simulink model "QuadcopterSimModel_INDI_Traj"  (R2018b)
settings: Solver=ode23  StartTime=0.0  StopTime=1000  FixedStep=sample_time  RelTol=1e-4  EnableMultiTasking=on
undefined symbols (not defined in the file): alt_ground, atmosphere, cycle, DiscIntNeverNeededParam, envir, fm_loiter, g, jystck, pos_ref, sigbuilder_block, traj_empty, waypoints, wind
libraries: simulink x6, ndi_lib x5, filters_lib x5, axes_transformation_lib x4, angles_lib x3, unit_conversions_lib x3, cntrl_atti_red_indi_lib x2, traj_lib x2, aerolibfltsims x2, control_allocation_lib x1, sensors_lib x1, atmosphere_lib x1
(part 2 of 3)

== system QuadcopterSimModel_INDI_Traj/stick inputs/Signal builder/Signal Builder2 ==
  Demux : Demux  Tag=STV Demux  Outputs=1
  FromWs : FromWorkspace  Tag=STV FromWs  VariableName=tuvar  SampleTime=0
      SigBuilderData=|
      | common.afterFinalStr = 'Extrapolate'
      | common.sampleTime = 0
      | dataSet.timeRange = [0 10]
      | dataSet.name = 'Group 1'
      | sbobj.Groups.Name = 'Group 1'
      | sbobj.Groups.Signals.Name = 'Signal 1'
      | sbobj.Groups.Signals.XData = [0 2 2 6 8 10]
      | sbobj.Groups.Signals.YData = [0 0 -1 -1 0 0]
  Signal 1 : Outport  Tag=STV Outport
  wires:
  FromWs/1 -> Demux/1
  Demux/1 -> Signal 1/1

== system QuadcopterSimModel_INDI_Traj/stick inputs/Signal builder/Signal Builder3 ==
  Demux : Demux  Tag=STV Demux  Outputs=1
  FromWs : FromWorkspace  Tag=STV FromWs  VariableName=tuvar  SampleTime=0
      SigBuilderData=|
      | common.afterFinalStr = 'Extrapolate'
      | common.sampleTime = 0
      | dataSet.timeRange = [0 10]
      | dataSet.name = 'Group 1'
      | sbobj.Groups.Name = 'Group 1'
      | sbobj.Groups.Signals.Name = 'Signal 1'
      | sbobj.Groups.Signals.XData = [0 6 6 8 8 10]
      | sbobj.Groups.Signals.YData = [0 0 1 1 0 0]
  Signal 1 : Outport  Tag=STV Outport
  wires:
  Demux/1 -> Signal 1/1
  FromWs/1 -> Demux/1

== system QuadcopterSimModel_INDI_Traj/Controller INDI/Multicopter INDI Loiter Flight Mode/Delta attitude to stick commands/conversion to total attitude command ==
  Delta_q : Inport
  Delta_n_g : Inport  Port=2
  M_bg : Inport  Port=3
  Add : Sum
  DCM to quaternions : axes_transformation_lib/DCM to quaternions  SystemSampleTime=-1
      settings: SourceProductName=LADAC
  MATLAB Function : MATLAB Function  TreatAsAtomicUnit=on
  MATLAB Function1 : MATLAB Function  TreatAsAtomicUnit=on
  MATLAB Function4 : MATLAB Function  TreatAsAtomicUnit=on
  Scope : Scope  NumInputPorts=4
  quaternion to lean angles : Subsystem
  total reduced attitude command (quaternion) : MATLAB Function  TreatAsAtomicUnit=on
  lean_angle : Outport
  lean_direction_angle : Outport  Port=2
  wires:
  DCM to quaternions/1 -> total reduced attitude command (quaternion)/2(q_m)
  M_bg/1 -> MATLAB Function1/1(M_bg), DCM to quaternions/1
  quaternion to lean angles/1(phi) -> Scope/1
  total reduced attitude command (quaternion)/1(q_cmd) -> quaternion to lean angles/1(q_bg)
  Add/1 -> MATLAB Function/1(u)
  Delta_q/1 -> total reduced attitude command (quaternion)/1(q_e)
  MATLAB Function4/1(phi) -> lean_angle/1, Scope/3
  quaternion to lean angles/2(delta) -> Scope/2
  MATLAB Function4/2(delta) -> Scope/4, lean_direction_angle/1
  Delta_n_g/1 -> Add/1
  MATLAB Function1/1(n_g) -> Add/2
  MATLAB Function/1(y) -> MATLAB Function4/1(n_g)

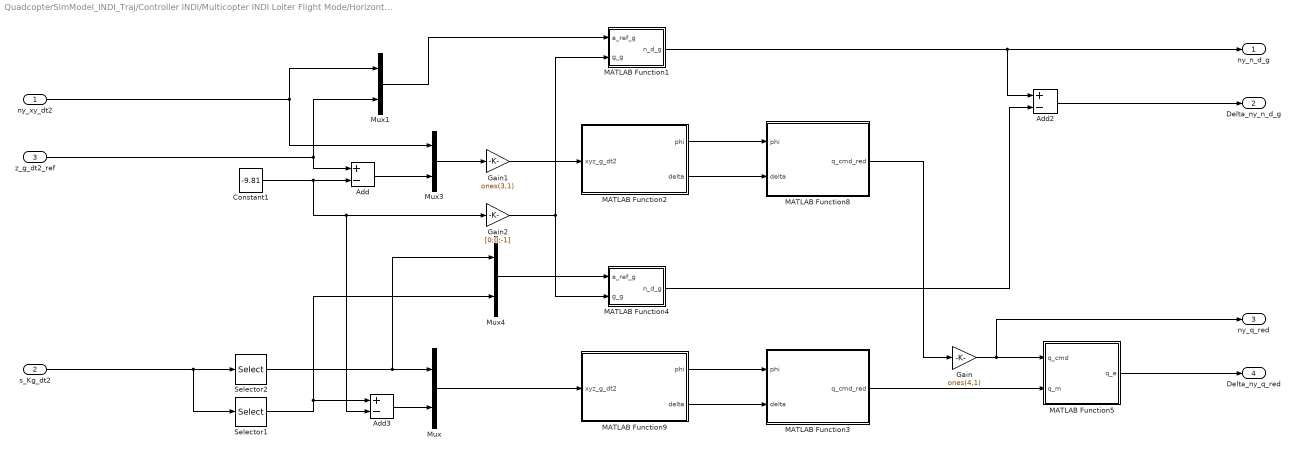
== system QuadcopterSimModel_INDI_Traj/Controller INDI/Multicopter INDI Loiter Flight Mode/Horizontal NDI position (NE) controller cascade with reduced attitude (angle) command/Convert to reduced attitude pseudo control ==
  ny_xy_dt2 : Inport
  s_Kg_dt2 : Inport  Port=2
  z_g_dt2_ref : Inport  Port=3
  Add : Sum  Inputs=+-
  Add2 : Sum  Inputs=+-
  Add3 : Sum  Inputs=+-
  Constant1 : Constant  Value=-9.81  OutDataTypeStr=single
  Gain : Gain  Gain=ones(4,1)
  Gain1 : Gain  Gain=ones(3,1)
  Gain2 : Gain  Gain=[0;0;-1]
  MATLAB Function1 : MATLAB Function  TreatAsAtomicUnit=on
  MATLAB Function2 : MATLAB Function  TreatAsAtomicUnit=on
  MATLAB Function3 : MATLAB Function  TreatAsAtomicUnit=on
  MATLAB Function4 : MATLAB Function  TreatAsAtomicUnit=on
  MATLAB Function5 : MATLAB Function  TreatAsAtomicUnit=on
  MATLAB Function8 : MATLAB Function  TreatAsAtomicUnit=on
  MATLAB Function9 : MATLAB Function  TreatAsAtomicUnit=on
  Mux{,1,3..4} (4 alike) : Mux  Inputs=2
  Selector1 : Selector  InputPortWidth=3  IndexOptions=Index vector (dialog)  Indices=3  OutputSizes=1
  Selector2 : Selector  InputPortWidth=3  IndexOptions=Index vector (dialog)  Indices=[1,2]  OutputSizes=1
  ny_n_d_g : Outport
  Delta_ny_n_d_g : Outport  Port=2
  ny_q_red : Outport  Port=3
  Delta_ny_q_red : Outport  Port=4
  wires:
  MATLAB Function2/1(phi) -> MATLAB Function8/1(phi)
  MATLAB Function8/1(q_cmd_red) -> Gain/1
  Gain/1 -> MATLAB Function5/1(q_cmd), ny_q_red/1
  MATLAB Function1/1(n_d_g) -> Add2/1, ny_n_d_g/1
  Constant1/1 -> Add3/2, Gain2/1, Add/2
  Mux3/1 -> Gain1/1
  ny_xy_dt2/1 -> Mux1/1, Mux3/1
  Mux1/1 -> MATLAB Function1/1(a_ref_g)
  MATLAB Function5/1(q_e) -> Delta_ny_q_red/1
  MATLAB Function9/1(phi) -> MATLAB Function3/1(phi)
  Gain2/1 -> MATLAB Function4/2(g_g), MATLAB Function1/2(g_g)
  Mux4/1 -> MATLAB Function4/1(a_ref_g)
  Add2/1 -> Delta_ny_n_d_g/1
  z_g_dt2_ref/1 -> Mux1/2, Add/1
  Gain1/1 -> MATLAB Function2/1(xyz_g_dt2)
  Add/1 -> Mux3/2
  MATLAB Function9/2(delta) -> MATLAB Function3/2(delta)
  s_Kg_dt2/1 -> Selector2/1, Selector1/1
  Add3/1 -> Mux/2
  Selector2/1 -> Mux4/1, Mux/1
  MATLAB Function4/1(n_d_g) -> Add2/2
  Selector1/1 -> Add3/1, Mux4/2
  MATLAB Function3/1(q_cmd_red) -> MATLAB Function5/2(q_m)
  MATLAB Function2/2(delta) -> MATLAB Function8/2(delta)
  Mux/1 -> MATLAB Function9/1(xyz_g_dt2)

== system QuadcopterSimModel_INDI_Traj/Controller INDI/Multicopter INDI Loiter Flight Mode/Horizontal NDI position (NE) controller cascade with reduced attitude (angle) command/filtered command ==
  cmd_forward_velocity_-1_1 : Inport
  cmd_lateral_velocity_-1_1 : Inport  Port=2
  initial_horizontal_position : Inport  Port=3
  manual_mode : Inport  Port=4
  Bus Creator : BusCreator  Inputs=3
  Bus Selector2 : BusSelector  OutputSignals=x_ref,x_dt_ref
  Discrete-Time Integrator : DiscreteIntegrator  ExternalReset=rising  InitialConditionSource=external  SampleTime=-1  ICPrevOutput=DiscIntNeverNeededParam  ICPrevScaledInput=DiscIntNeverNeededParam
  Gain : Gain
  Gain1 : Gain
  Gain3 : Gain  Gain=horiz_pos_cntrl.rm.uv_max
  MATLAB Function1 : MATLAB Function  TreatAsAtomicUnit=on
  Mux : Mux  Inputs=2
  PT1 discrete reference model : ndi_lib/PT1 discrete reference model  T=horiz_pos_cntrl.rm.uv_T  x_max=inf  x_min=-inf  x_dt_max=horiz_pos_cntrl.rm.uv_dt_max  x_dt_min=-horiz_pos_cntrl.rm.uv_dt_max  x_init=0
      settings: SourceProductName=LADAC
  Product : Product
  Terminator : Terminator
  ny : Outport
  reference : Outport  Port=2
  wires:
  Gain3/1 -> Product/2
  Product/1 -> PT1 discrete reference model/1
  MATLAB Function1/1(cmd_velocity_abs_0_1) -> Gain3/1
  MATLAB Function1/2(lean_direction_angle) -> Terminator/1
  Mux/1 -> Product/1
  Gain1/1 -> Bus Creator/3, ny/1  "xy_g_dt2"
  Gain/1 -> Bus Creator/2  "xy_g_dt"
  cmd_lateral_velocity_-1_1/1 -> MATLAB Function1/1(stick_roll_cmd), Mux/2
  initial_horizontal_position/1 -> Discrete-Time Integrator/3
  Bus Selector2/2 -> Gain1/1  "<x_dt_ref>"
  Bus Selector2/1 -> Discrete-Time Integrator/1, Gain/1  "<x_ref>"
  Discrete-Time Integrator/1 -> Bus Creator/1  "xy_g"
  PT1 discrete reference model/1 -> Bus Selector2/1
  Bus Creator/1 -> reference/1
  cmd_forward_velocity_-1_1/1 -> MATLAB Function1/2(stick_pitch_cmd), Mux/1
  manual_mode/1 -> Discrete-Time Integrator/2

== system QuadcopterSimModel_INDI_Traj/Controller INDI/Multicopter INDI Loiter Flight Mode/Horizontal NDI position (NE) controller cascade with reduced attitude (angle) command/measures ==
  xy_g : Inport
  xy_g_dt : Inport  Port=2
  s_Kg_dt2 : Inport  Port=3
  Bus Creator1 : BusCreator  Inputs=4
  Selector3 : Selector  InputPortWidth=3  IndexOptions=Index vector (dialog)  Indices=[1,2]  OutputSizes=1
  Selector4 : Selector  InputPortWidth=3  IndexOptions=Index vector (dialog)  Indices=[1,2]  OutputSizes=1
  Selector5 : Selector  InputPortWidth=3  IndexOptions=Index vector (dialog)  Indices=[1,2]  OutputSizes=1
  Selector6 : Selector  InputPortWidth=3  IndexOptions=Index vector (dialog)  Indices=3  OutputSizes=1
  measure : Outport
  wires:
  s_Kg_dt2/1 -> Selector6/1, Selector5/1
  xy_g_dt/1 -> Selector4/1
  xy_g/1 -> Selector3/1
  Selector4/1 -> Bus Creator1/2  "xy_g_dt"
  Selector3/1 -> Bus Creator1/1  "xy_g"
  Selector5/1 -> Bus Creator1/3  "xy_g_dt2"
  Selector6/1 -> Bus Creator1/4  "z_g_dt2"
  Bus Creator1/1 -> measure/1

== system QuadcopterSimModel_INDI_Traj/Controller INDI/Multicopter INDI Loiter Flight Mode/Horizontal NDI position (NE) controller cascade with reduced attitude (angle) command/position controller ==
  reference : Inport
  measure : Inport  Port=2
  Add : Sum  Inputs=+-
  Bus Selector : BusSelector  OutputSignals=xy_g,xy_g_dt,xy_g_dt2
  Bus to Vector : BusToVector
  Gain : Gain  Gain=horiz_pos_cntrl.K  Multiplication=Matrix(K*u)
  Mux : Mux  Inputs=3
  PT2 discrete with saturation : filters_lib/PT2 discrete with saturation  omega=2./T  d=1  x_dt2_max=inf  x_dt2_min=-inf  x_dt_max=inf  x_dt_min=-inf  x_max=inf  x_min=-inf  x_init=0  x_dt_init=0
      settings: SourceProductName=LADAC
  Saturation : Saturate  UpperLimit=horiz_pos_cntrl.limits.uv_dt_max  LowerLimit=-horiz_pos_cntrl.limits.uv_dt_max
  Saturation1 : Saturate  UpperLimit=[horiz_pos_cntrl.limits.e_xy_max;1000;1000;1000;1000]  LowerLimit=-[horiz_pos_cntrl.limits.e_xy_max;1000;1000;1000;1000]
  Terminator : Terminator
  Terminator1 : Terminator
  ny_cntrl : Outport
  e : Outport  Port=2
  wires:
  PT2 discrete with saturation/1 -> Add/1
  PT2 discrete with saturation/3 -> Terminator1/1
  PT2 discrete with saturation/2 -> Terminator/1
  Bus to Vector/1 -> PT2 discrete with saturation/1
  Bus Selector/1 -> Mux/1  "<xy_g>"
  Bus Selector/2 -> Mux/2  "<xy_g_dt>"
  Bus Selector/3 -> Mux/3  "<xy_g_dt2>"
  Mux/1 -> Add/2
  measure/1 -> Bus Selector/1
  Gain/1 -> Saturation/1
  Saturation1/1 -> Gain/1
  Saturation/1 -> ny_cntrl/1
  Add/1 -> e/1, Saturation1/1
  reference/1 -> Bus to Vector/1

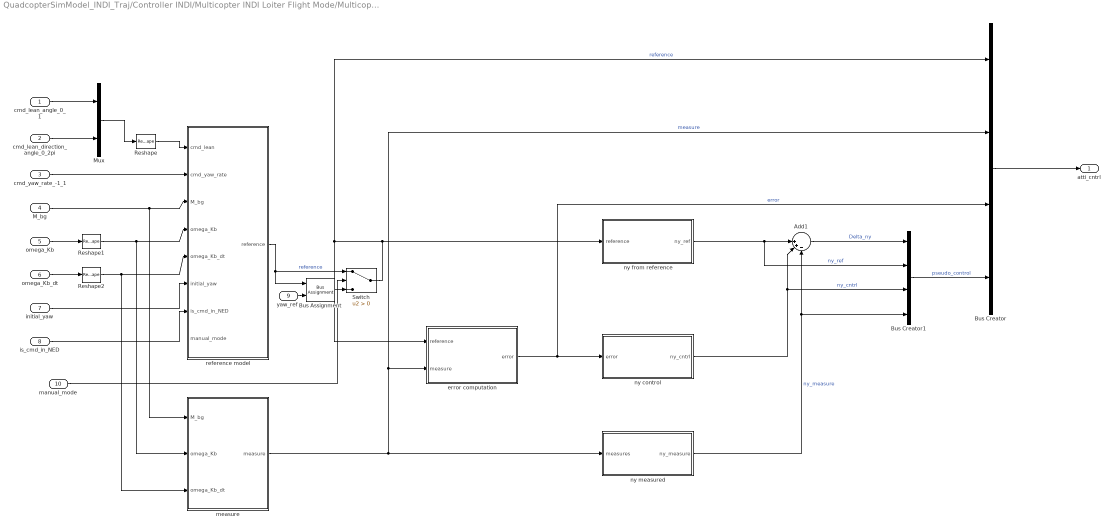
== system QuadcopterSimModel_INDI_Traj/Controller INDI/Multicopter INDI Loiter Flight Mode/Multicopter Altitude Hold Flight Mode with INDI and reduced attitude control/Multicopter (Reduced) Attitude INDI Controller ==
  cmd_lean_angle_0_1 : Inport
  cmd_lean_direction_angle_0_2pi : Inport  Port=2
  cmd_yaw_rate_-1_1 : Inport  Port=3
  M_bg : Inport  Port=4
  omega_Kb : Inport  Port=5
  omega_Kb_dt : Inport  Port=6
  initial_yaw : Inport  Port=7
  is_cmd_in_NED : Inport  Port=8
  "yaw_ref " : Inport  Port=9
  manual_mode : Inport  Port=10
  Add1 : Sum  Inputs=||++-
  Bus Assignment : BusAssignment  AssignedSignals=yaw
  Bus Creator : BusCreator  Inputs=4
  Bus Creator1 : BusCreator  Inputs=4
  Mux : Mux  Inputs=2
  Reshape : Reshape  OutputDimensionality=Column vector (2-D)
  Reshape1 : Reshape  OutputDimensionality=Column vector (2-D)
  Reshape2 : Reshape  OutputDimensionality=Column vector (2-D)
  Switch : Switch  Criteria=u2 > Threshold
  error computation : Subsystem
  measure : Subsystem
  ny control : Subsystem
  ny from reference : Subsystem
  ny measured : Subsystem
  reference model : Subsystem
  atti_cntrl : Outport
  wires:
  is_cmd_in_NED/1 -> reference model/7(is_cmd_in_NED)
  cmd_yaw_rate_-1_1/1 -> reference model/2(cmd_yaw_rate)
  cmd_lean_direction_angle_0_2pi/1 -> Mux/2
  cmd_lean_angle_0_1/1 -> Mux/1
  Reshape2/1 -> reference model/5(omega_Kb_dt), measure/3(omega_Kb_dt)
  Reshape1/1 -> reference model/4(omega_Kb), measure/2(omega_Kb)
  Reshape/1 -> reference model/1(cmd_lean)
  measure/1(measure) -> ny measured/1(measures), error computation/2(measure), Bus Creator/2  "measure"
  omega_Kb/1 -> Reshape1/1
  M_bg/1 -> reference model/3(M_bg), measure/1(M_bg)
  Add1/1 -> Bus Creator1/1  "Delta_ny"
  Bus Creator1/1 -> Bus Creator/4  "pseudo_control"
  Bus Creator/1 -> atti_cntrl/1
  initial_yaw/1 -> reference model/6(initial_yaw)
  Switch/1 -> error computation/1(reference), Bus Creator/1, ny from reference/1(reference)  "reference"
  ny measured/1(ny_measure) -> Add1/3, Bus Creator1/4  "ny_measure"
  ny control/1(ny_cntrl) -> Add1/2, Bus Creator1/3  "ny_cntrl"
  omega_Kb_dt/1 -> Reshape2/1
  error computation/1(error) -> Bus Creator/3, ny control/1(error)  "error"
  Mux/1 -> Reshape/1
  ny from reference/1(ny_ref) -> Add1/1, Bus Creator1/2  "ny_ref"
  manual_mode/1 -> Switch/2
  "yaw_ref "/1 -> Bus Assignment/2
  reference model/1(reference) -> Switch/1, Bus Assignment/1  "reference"
  Bus Assignment/1 -> Switch/3

== system QuadcopterSimModel_INDI_Traj/Controller INDI/Multicopter INDI Loiter Flight Mode/Multicopter Altitude Hold Flight Mode with INDI and reduced attitude control/Multicopter Altitude INDI Controller1 ==
  cmd_throttle_-1_1 : Inport
  z_Kg : Inport  Port=2
  z_Kg_dt : Inport  Port=3
  z_Kg_dt2 : Inport  Port=4
  initial_z_Kg : Inport  Port=5
  z_Ref : Inport  Port=6
  manual_mode : Inport  Port=7
  Add1 : Sum  Inputs=||++-
  Bus Creator : BusCreator  Inputs=4
  Bus Creator1 : BusCreator  Inputs=4
  Switch : Switch  Criteria=u2 > Threshold
  error computation : Subsystem
  measure : Subsystem
  ny control : Subsystem
  ny from reference : Subsystem
  ny measured : Subsystem
  reference model : Subsystem
  alt_cntrl : Outport
  wires:
  cmd_throttle_-1_1/1 -> reference model/1(cmd_throttle)
  z_Kg/1 -> measure/1(z_Kg)
  z_Kg_dt/1 -> measure/2(z_Kg_dt)
  z_Kg_dt2/1 -> measure/3(z_Kg_dt2)
  measure/1(measure) -> error computation/2(measure), Bus Creator/2, ny measured/1(measures)  "measure"
  Add1/1 -> Bus Creator1/1  "Delta_ny"
  Bus Creator1/1 -> Bus Creator/4  "pseudo_control"
  Bus Creator/1 -> alt_cntrl/1
  initial_z_Kg/1 -> reference model/2(initial_altitude)
  Switch/1 -> Bus Creator/1, ny from reference/1(reference_alt), error computation/1(reference)  "reference"
  ny measured/1(ny_measure) -> Add1/3, Bus Creator1/4  "ny_measure"
  ny control/1(ny_cntrl) -> Add1/2, Bus Creator1/3  "ny_cntrl"
  error computation/1(error) -> Bus Creator/3, ny control/1(error_alt)  "error"
  ny from reference/1(ny_ref) -> Add1/1, Bus Creator1/2  "ny_ref"
  z_Ref/1 -> Switch/3  "reference"
  reference model/1(reference) -> Switch/1  "reference"
  manual_mode/1 -> Switch/2, reference model/3(manual_mode)

== system QuadcopterSimModel_INDI_Traj/Controller INDI/Multicopter INDI Loiter Flight Mode/Multicopter Altitude Hold Flight Mode with INDI and reduced attitude control/acceleration g to b frame ==
  z_Kg_dt2_cmd : Inport
  M_bg : Inport  Port=2
  MATLAB Function : MATLAB Function  TreatAsAtomicUnit=on
  dcm2Lean : MATLAB Function  TreatAsAtomicUnit=on
  z_Kb_dt2_cmd : Outport
  wires:
  dcm2Lean/1(phi) -> MATLAB Function/2(lean_angle)
  M_bg/1 -> dcm2Lean/1(M_bg)
  MATLAB Function/1(z_Kb_dt2_cmd) -> z_Kb_dt2_cmd/1
  z_Kg_dt2_cmd/1 -> MATLAB Function/1(z_Kg_dt2_cmd)

== system QuadcopterSimModel_INDI_Traj/Controller INDI/Multicopter INDI Loiter Flight Mode/Multicopter Altitude Hold Flight Mode with INDI and reduced attitude control/control effectiveness ==
  u : Inport
  Constant : Constant  Value=fm.cntrl_effect.u_trim  OutDataTypeStr=single
  Constant1 : Constant  Value=fm.ca.u_min  OutDataTypeStr=single
  Constant4 : Constant  Value=fm.sample_time  OutDataTypeStr=single
  MATLAB Function : MATLAB Function  TreatAsAtomicUnit=on
  Max : MinMax  Function=max  Inputs=2  OutDataTypeStr=Inherit: Inherit via back propagation
  ny_du_dt : Constant  Value=fm.cntrl_effect.ny_du_dt  OutDataTypeStr=single
  ny_du_red_trim : Constant  Value=fm.cntrl_effect.ny_du_red  OutDataTypeStr=single
  G1 : Outport
  G2 : Outport  Port=2
  wires:
  ny_du_red_trim/1 -> MATLAB Function/1(ny_du_red_trim)
  Constant4/1 -> MATLAB Function/5(T_s)
  Constant/1 -> MATLAB Function/3(u_trim)
  ny_du_dt/1 -> MATLAB Function/2(ny_du_dt_trim)
  u/1 -> Max/1
  Constant1/1 -> Max/2
  Max/1 -> MATLAB Function/4(u)
  MATLAB Function/1(G1) -> G1/1
  MATLAB Function/2(G2) -> G2/1

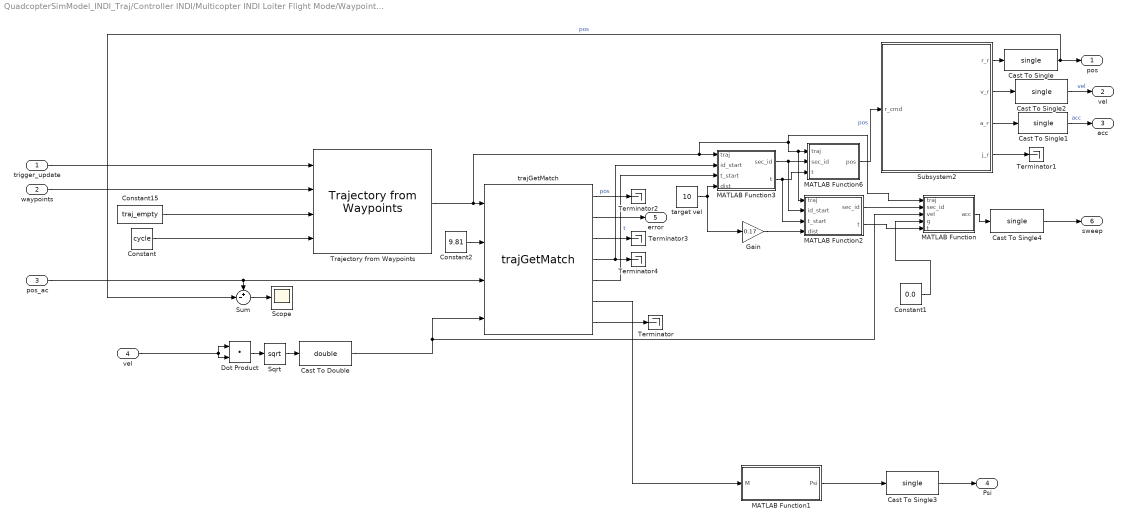
== system QuadcopterSimModel_INDI_Traj/Controller INDI/Multicopter INDI Loiter Flight Mode/Waypoint Reference/waypoint Reference System ==
  trigger_update : Inport
  waypoints : Inport  Port=2
  pos_ac : Inport  Port=3
  "vel " : Inport  Port=4
  Cast To Double : DataTypeConversion  OutDataTypeStr=double
  Cast To Single{,1..4} (5 alike) : DataTypeConversion  OutDataTypeStr=single
  Constant : Constant  Value=cycle
  Constant1 : Constant  Value=0.0
  Constant15 : Constant  Value=traj_empty  OutDataTypeStr=Bus: trajectoryBus
  Constant2 : Constant  Value=9.81
  Dot Product : DotProduct  InputSameDT=on  OutDataTypeStr=Inherit: Inherit via internal rule
  Gain : Gain  Gain=0.17
  MATLAB Function : MATLAB Function  TreatAsAtomicUnit=on
  MATLAB Function1 : MATLAB Function  TreatAsAtomicUnit=on
  MATLAB Function2 : MATLAB Function  TreatAsAtomicUnit=on
  MATLAB Function3 : MATLAB Function  TreatAsAtomicUnit=on
  MATLAB Function6 : MATLAB Function  TreatAsAtomicUnit=on
  Scope : Scope
  Sqrt : Sqrt  SaturateOnIntegerOverflow=on
  Subsystem2 : Subsystem
  Sum : Sum  Inputs=+-|
  Terminator{,1..4} (5 alike) : Terminator
  Trajectory from Waypoints : traj_lib/Trajectory from Waypoints
      settings: SourceProductName=LADAC
  target vel : Constant  Value=10
  trajGetMatch : traj_lib/trajGetMatch  SystemSampleTime=-1
      settings: SourceProductName=LADAC
  pos : Outport
  vel : Outport  Port=2
  acc : Outport  Port=3
  Psi : Outport  Port=4
  error : Outport  Port=5
  "sweep " : Outport  Port=6
  wires:
  Constant15/1 -> Trajectory from Waypoints/3
  waypoints/1 -> Trajectory from Waypoints/2
  trajGetMatch/4 -> MATLAB Function3/2(id_start), Terminator4/1
  "vel "/1 -> Dot Product/2, Dot Product/1
  Cast To Single1/1 -> acc/1  "acc"
  pos_ac/1 -> trajGetMatch/3, Sum/1
  Cast To Single2/1 -> vel/1  "vel"
  Cast To Single/1 -> Sum/2, pos/1  "pos"
  trajGetMatch/3 -> Terminator3/1
  Constant/1 -> Trajectory from Waypoints/4
  Constant2/1 -> trajGetMatch/2
  trajGetMatch/6 -> MATLAB Function1/1(M)
  trajGetMatch/5 -> MATLAB Function3/3(t_start)  "t"
  trigger_update/1 -> Trajectory from Waypoints/1
  trajGetMatch/2 -> error/1
  Cast To Single3/1 -> Psi/1
  MATLAB Function1/1(Psi) -> Cast To Single3/1
  Sum/1 -> Scope/1
  Dot Product/1 -> Sqrt/1
  Cast To Double/1 -> MATLAB Function/3(vel), trajGetMatch/4
  MATLAB Function3/1(sec_id) -> MATLAB Function2/2(id_start), MATLAB Function6/2(sec_id)
  Subsystem2/1(r_r) -> Cast To Single/1
  Subsystem2/2(v_r) -> Cast To Single2/1
  Subsystem2/3(a_r) -> Cast To Single1/1
  trajGetMatch/1 -> Terminator2/1  "pos"
  MATLAB Function6/1(pos) -> Subsystem2/1(r_cmd)  "pos"
  target vel/1 -> MATLAB Function3/4(dist), Gain/1
  Sqrt/1 -> Cast To Double/1
  trajGetMatch/7 -> Terminator/1
  Subsystem2/4(j_r) -> Terminator1/1
  MATLAB Function3/2(t) -> MATLAB Function2/3(t_start), MATLAB Function6/3(t)
  Gain/1 -> MATLAB Function2/4(dist)
  MATLAB Function2/2(t) -> MATLAB Function/5(t)
  MATLAB Function2/1(sec_id) -> MATLAB Function/2(sec_id)
  Constant1/1 -> MATLAB Function/4(g)
  MATLAB Function/1(acc) -> Cast To Single4/1
  Cast To Single4/1 -> "sweep "/1
  Trajectory from Waypoints/1 -> MATLAB Function/1(traj), MATLAB Function2/1(traj), MATLAB Function6/1(traj), MATLAB Function3/1(traj), trajGetMatch/1

== system QuadcopterSimModel_INDI_Traj/Controller INDI/Multicopter INDI Loiter Flight Mode/Delta attitude to stick commands/conversion to total attitude command/quaternion to lean angles ==
  q_bg : Inport
  MATLAB Function4 : MATLAB Function  TreatAsAtomicUnit=on
  quaternion to reduced attitude unit vector : MATLAB Function  TreatAsAtomicUnit=on
  phi : Outport
  delta : Outport  Port=2
  wires:
  MATLAB Function4/2(delta) -> delta/1
  q_bg/1 -> quaternion to reduced attitude unit vector/1(q_bg)
  MATLAB Function4/1(phi) -> phi/1
  quaternion to reduced attitude unit vector/1(n_g) -> MATLAB Function4/1(n_g)

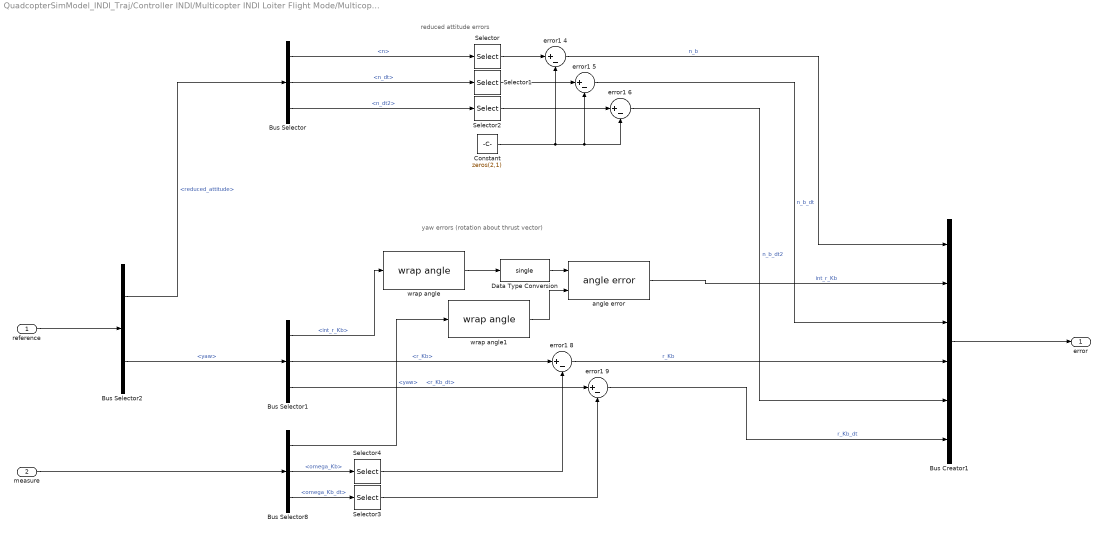
== system QuadcopterSimModel_INDI_Traj/Controller INDI/Multicopter INDI Loiter Flight Mode/Multicopter Altitude Hold Flight Mode with INDI and reduced attitude control/Multicopter (Reduced) Attitude INDI Controller/error computation ==
  note: yaw errors (rotation about thrust vector)
  note: reduced attitude errors
  reference : Inport
  measure : Inport  Port=2
  Bus Creator1 : BusCreator  Inputs=6
  Bus Selector : BusSelector  OutputSignals=n,n_dt,n_dt2
  Bus Selector1 : BusSelector  OutputSignals=int_r_Kb,r_Kb,r_Kb_dt
  Bus Selector2 : BusSelector  OutputSignals=reduced_attitude,yaw
  Bus Selector8 : BusSelector  OutputSignals=yaw,omega_Kb,omega_Kb_dt
  Constant : Constant  Value=zeros(2,1)  OutDataTypeStr=Inherit: Inherit via back propagation
  Data Type Conversion : DataTypeConversion  OutDataTypeStr=single
  Selector : Selector  InputPortWidth=3  IndexOptions=Index vector (dialog)  Indices=[1,2]  OutputSizes=1
  Selector1 : Selector  InputPortWidth=3  IndexOptions=Index vector (dialog)  Indices=[1,2]  OutputSizes=1
  Selector2 : Selector  InputPortWidth=3  IndexOptions=Index vector (dialog)  Indices=[1,2]  OutputSizes=1
  Selector3 : Selector  InputPortWidth=3  IndexOptions=Index vector (dialog)  Indices=3  OutputSizes=1
  Selector4 : Selector  InputPortWidth=3  IndexOptions=Index vector (dialog)  Indices=3  OutputSizes=1
  angle error : angles_lib/angle error  SystemSampleTime=-1
      settings: SourceProductName=LADAC
  error1 {4..6,8..9} (5 alike) : Sum  Inputs=|+-
  wrap angle : angles_lib/wrap angle  SystemSampleTime=-1
      settings: SourceProductName=LADAC
  wrap angle1 : angles_lib/wrap angle  SystemSampleTime=-1
      settings: SourceProductName=LADAC
  error : Outport
  wires:
  Data Type Conversion/1 -> angle error/1
  wrap angle/1 -> Data Type Conversion/1
  wrap angle1/1 -> angle error/2
  error1 9/1 -> Bus Creator1/6  "r_Kb_dt"
  error1 6/1 -> Bus Creator1/5  "n_b_dt2"
  error1 5/1 -> Bus Creator1/3  "n_b_dt"
  error1 8/1 -> Bus Creator1/4  "r_Kb"
  angle error/1 -> Bus Creator1/2  "int_r_Kb"
  Selector3/1 -> error1 9/2
  Selector4/1 -> error1 8/2
  Bus Selector8/1 -> wrap angle1/1  "<yaw>"
  Bus Selector8/2 -> Selector4/1  "<omega_Kb>"
  Bus Selector8/3 -> Selector3/1  "<omega_Kb_dt>"
  measure/1 -> Bus Selector8/1
  Bus Selector1/3 -> error1 9/1  "<r_Kb_dt>"
  Bus Selector1/2 -> error1 8/1  "<r_Kb>"
  Bus Selector1/1 -> wrap angle/1  "<int_r_Kb>"
  Bus Selector2/2 -> Bus Selector1/1  "<yaw>"
  Constant/1 -> error1 4/2, error1 5/2, error1 6/2
  Selector2/1 -> error1 6/1
  Selector1/1 -> error1 5/1
  Selector/1 -> error1 4/1
  Bus Creator1/1 -> error/1
  Bus Selector2/1 -> Bus Selector/1  "<reduced_attitude>"
  Bus Selector/3 -> Selector2/1  "<n_dt2>"
  Bus Selector/2 -> Selector1/1  "<n_dt>"
  Bus Selector/1 -> Selector/1  "<n>"
  reference/1 -> Bus Selector2/1
  error1 4/1 -> Bus Creator1/1  "n_b"

== system QuadcopterSimModel_INDI_Traj/Controller INDI/Multicopter INDI Loiter Flight Mode/Multicopter Altitude Hold Flight Mode with INDI and reduced attitude control/Multicopter (Reduced) Attitude INDI Controller/measure ==
  M_bg : Inport
  omega_Kb : Inport  Port=2
  omega_Kb_dt : Inport  Port=3
  Bus Creator2 : BusCreator  Inputs=3
  DCM to quaternions : axes_transformation_lib/DCM to quaternions  SystemSampleTime=-1
      settings: SourceProductName=LADAC
  MATLAB Function1 : MATLAB Function  TreatAsAtomicUnit=on
  Terminator : Terminator
  measure : Outport
  wires:
  Bus Creator2/1 -> measure/1  "measure"
  omega_Kb_dt/1 -> Bus Creator2/3  "omega_Kb_dt"
  omega_Kb/1 -> Bus Creator2/2  "omega_Kb"
  M_bg/1 -> DCM to quaternions/1
  MATLAB Function1/2(yaw) -> Bus Creator2/1  "yaw"
  MATLAB Function1/1(q_red) -> Terminator/1
  DCM to quaternions/1 -> MATLAB Function1/1(q_bg)

== system QuadcopterSimModel_INDI_Traj/Controller INDI/Multicopter INDI Loiter Flight Mode/Multicopter Altitude Hold Flight Mode with INDI and reduced attitude control/Multicopter (Reduced) Attitude INDI Controller/ny control ==
  error : Inport
  Bus to Vector : BusToVector
  Gain : Gain  Gain=atti_cntrl.K  Multiplication=Matrix(K*u)
  ny_cntrl : Outport
  wires:
  Bus to Vector/1 -> Gain/1
  error/1 -> Bus to Vector/1
  Gain/1 -> ny_cntrl/1

== system QuadcopterSimModel_INDI_Traj/Controller INDI/Multicopter INDI Loiter Flight Mode/Multicopter Altitude Hold Flight Mode with INDI and reduced attitude control/Multicopter (Reduced) Attitude INDI Controller/ny from reference ==
  reference : Inport
  Bus Selector2 : BusSelector  OutputSignals=reduced_attitude.ny_n_dt2,yaw.r_Kb_dt
  Mux2 : Mux  Inputs=2
  Selector : Selector  InputPortWidth=3  IndexOptions=Index vector (dialog)  Indices=[1,2]  OutputSizes=1
  ny_ref : Outport
  wires:
  Selector/1 -> Mux2/1
  Bus Selector2/1 -> Selector/1  "<ny_n_dt2>"
  Bus Selector2/2 -> Mux2/2  "<r_Kb_dt>"
  Mux2/1 -> ny_ref/1
  reference/1 -> Bus Selector2/1

== system QuadcopterSimModel_INDI_Traj/Controller INDI/Multicopter INDI Loiter Flight Mode/Multicopter Altitude Hold Flight Mode with INDI and reduced attitude control/Multicopter (Reduced) Attitude INDI Controller/ny measured ==
  measures : Inport
  Bus Selector2 : BusSelector  OutputSignals=omega_Kb_dt
  Constant1 : Constant  Value=zeros(2,1)  OutDataTypeStr=Inherit: Inherit via back propagation
  Mux1 : Mux  Inputs=2
  Selector2 : Selector  InputPortWidth=3  IndexOptions=Index vector (dialog)  Indices=3  OutputSizes=1
  ny_measure : Outport
  wires:
  Constant1/1 -> Mux1/1
  Selector2/1 -> Mux1/2
  Mux1/1 -> ny_measure/1
  measures/1 -> Bus Selector2/1
  Bus Selector2/1 -> Selector2/1  "<omega_Kb_dt>"

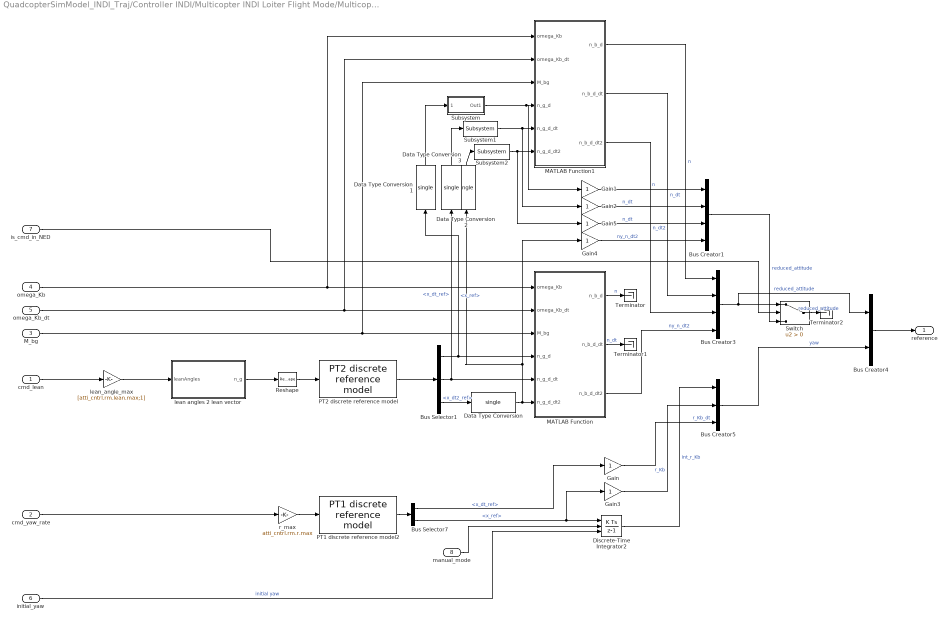
== system QuadcopterSimModel_INDI_Traj/Controller INDI/Multicopter INDI Loiter Flight Mode/Multicopter Altitude Hold Flight Mode with INDI and reduced attitude control/Multicopter (Reduced) Attitude INDI Controller/reference model ==
  cmd_lean : Inport
  cmd_yaw_rate : Inport  Port=2
  M_bg : Inport  Port=3
  omega_Kb : Inport  Port=4
  omega_Kb_dt : Inport  Port=5
  initial_yaw : Inport  Port=6
  is_cmd_in_NED : Inport  Port=7
  manual_mode : Inport  Port=8
  Bus Creator1 : BusCreator  Inputs=4
  Bus Creator3 : BusCreator  Inputs=4
  Bus Creator4 : BusCreator  Inputs=2
  Bus Creator5 : BusCreator  Inputs=3
  Bus Selector1 : BusSelector  OutputSignals=x_ref,x_dt_ref,x_dt2_ref
  Bus Selector7 : BusSelector  OutputSignals=x_dt_ref,x_ref
  Data Type Conversion{,1..3} (4 alike) : DataTypeConversion  OutDataTypeStr=single
  Discrete-Time Integrator2 : DiscreteIntegrator  ExternalReset=rising  InitialConditionSource=external  SampleTime=-1  ICPrevOutput=DiscIntNeverNeededParam  ICPrevScaledInput=DiscIntNeverNeededParam
  Gain{,1..5} (6 alike) : Gain
  MATLAB Function : MATLAB Function  TreatAsAtomicUnit=on
  MATLAB Function1 : MATLAB Function  TreatAsAtomicUnit=on
  PT1 discrete reference model2 : ndi_lib/PT1 discrete reference model  T=atti_cntrl.rm.r.T  x_max=inf  x_min=-inf  x_dt_max=inf  x_dt_min=-inf  x_init=0
      settings: SourceProductName=LADAC
  PT2 discrete reference model : ndi_lib/PT2 discrete reference model  omega=atti_cntrl.rm.lean.omega  d=atti_cntrl.rm.lean.D  x_dt2_max=inf  x_dt2_min=-inf  x_dt_max=inf  x_dt_min=-inf  x_max=inf  x_min=-inf  x_init=single([0;0;-1])  x_dt_init=0
      settings: SourceProductName=LADAC
  Reshape : Reshape  OutputDimensionality=Column vector (2-D)
  Subsystem : Subsystem
  Subsystem1 : cntrl_atti_red_indi_lib/Multicopter (Reduced) Attitude INDI Controller/reference model/Subsystem  SystemSampleTime=-1
      settings: SourceProductName=LADAC
  Subsystem2 : cntrl_atti_red_indi_lib/Multicopter (Reduced) Attitude INDI Controller/reference model/Subsystem  SystemSampleTime=-1
      settings: SourceProductName=LADAC
  Switch : Switch  Criteria=u2 > Threshold
  Terminator : Terminator
  Terminator1 : Terminator
  Terminator2 : Terminator
  lean angles 2 lean vector : MATLAB Function  TreatAsAtomicUnit=on
  lean_angle_max : Gain  Gain=[atti_cntrl.rm.lean.max;1]
  r_max : Gain  Gain=atti_cntrl.rm.r.max
  reference : Outport
  wires:
  Subsystem2/1 -> MATLAB Function1/6(n_g_d_dt2), Gain5/1
  Subsystem1/1 -> Gain2/1, MATLAB Function1/5(n_g_d_dt)
  Subsystem/1(Out1) -> MATLAB Function1/4(n_g_d), Gain1/1
  Switch/1 -> Terminator2/1  "reduced_attitude"
  Gain5/1 -> Bus Creator1/3  "n_dt"
  MATLAB Function/2(n_b_d_dt) -> Terminator1/1  "n_dt"
  MATLAB Function/1(n_b_d) -> Terminator/1  "n"
  MATLAB Function1/3(n_b_d_dt2) -> Bus Creator3/3  "n_dt2"
  Data Type Conversion2/1 -> Subsystem2/1
  Data Type Conversion3/1 -> Subsystem1/1
  Data Type Conversion1/1 -> Subsystem/1(<x_ref>)
  lean_angle_max/1 -> lean angles 2 lean vector/1(leanAngles)
  Gain4/1 -> Bus Creator1/4  "ny_n_dt2"
  Gain2/1 -> Bus Creator1/2  "n_dt"
  Gain1/1 -> Bus Creator1/1  "n"
  is_cmd_in_NED/1 -> Switch/2
  Bus Creator1/1 -> Switch/3  "reduced_attitude"
  Reshape/1 -> PT2 discrete reference model/1
  cmd_lean/1 -> lean_angle_max/1
  Data Type Conversion/1 -> Data Type Conversion2/1, Gain4/1, MATLAB Function/6(n_g_d_dt2)
  Gain3/1 -> Bus Creator5/2  "r_Kb"
  Gain/1 -> Bus Creator5/3  "r_Kb_dt"
  Discrete-Time Integrator2/1 -> Bus Creator5/1  "int_r_Kb"
  Bus Creator5/1 -> Bus Creator4/2  "yaw"
  Bus Selector7/2 -> Discrete-Time Integrator2/1, Gain3/1  "<x_ref>"
  PT1 discrete reference model2/1 -> Bus Selector7/1
  Bus Selector7/1 -> Gain/1  "<x_dt_ref>"
  r_max/1 -> PT1 discrete reference model2/1
  cmd_yaw_rate/1 -> r_max/1
  M_bg/1 -> MATLAB Function/3(M_bg), MATLAB Function1/3(M_bg)
  omega_Kb_dt/1 -> MATLAB Function/2(omega_Kb_dt), MATLAB Function1/2(omega_Kb_dt)
  omega_Kb/1 -> MATLAB Function/1(omega_Kb), MATLAB Function1/1(omega_Kb)
  Bus Creator3/1 -> Switch/1, Bus Creator4/1  "reduced_attitude"
  Bus Creator4/1 -> reference/1
  lean angles 2 lean vector/1(n_g) -> Reshape/1
  MATLAB Function1/1(n_b_d) -> Bus Creator3/1  "n"
  Bus Selector1/3 -> Data Type Conversion/1  "<x_dt2_ref>"
  Bus Selector1/2 -> Data Type Conversion3/1, MATLAB Function/5(n_g_d_dt)  "<x_dt_ref>"
  MATLAB Function1/2(n_b_d_dt) -> Bus Creator3/2  "n_dt"
  PT2 discrete reference model/1 -> Bus Selector1/1
  MATLAB Function/3(n_b_d_dt2) -> Bus Creator3/4  "ny_n_dt2"
  Bus Selector1/1 -> MATLAB Function/4(n_g_d), Data Type Conversion1/1  "<x_ref>"
  initial_yaw/1 -> Discrete-Time Integrator2/3  "initial yaw"
  manual_mode/1 -> Discrete-Time Integrator2/2

== system QuadcopterSimModel_INDI_Traj/Controller INDI/Multicopter INDI Loiter Flight Mode/Multicopter Altitude Hold Flight Mode with INDI and reduced attitude control/Multicopter Altitude INDI Controller1/error computation ==
  note: altitude errors
  reference : Inport
  measure : Inport  Port=2
  Bus Creator1 : BusCreator  Inputs=3
  Bus Selector4 : BusSelector  OutputSignals=z_Kg,z_Kg_dt,z_Kg_dt2
  Bus Selector5 : BusSelector  OutputSignals=z_Kg,z_Kg_dt,z_Kg_dt2
  error1 1 : Sum  Inputs=|+-
  error1 2 : Sum  Inputs=|+-
  error1 3 : Sum  Inputs=|+-
  error : Outport
  wires:
  Bus Creator1/1 -> error/1
  error1 2/1 -> Bus Creator1/3  "alt_dt2"
  error1 1/1 -> Bus Creator1/2  "alt_dt"
  error1 3/1 -> Bus Creator1/1  "alt"
  Bus Selector5/1 -> error1 3/2  "<z_Kg>"
  Bus Selector4/1 -> error1 3/1  "<z_Kg>"
  Bus Selector5/3 -> error1 2/2  "<z_Kg_dt2>"
  Bus Selector4/3 -> error1 2/1  "<z_Kg_dt2>"
  measure/1 -> Bus Selector5/1
  reference/1 -> Bus Selector4/1
  Bus Selector5/2 -> error1 1/2  "<z_Kg_dt>"
  Bus Selector4/2 -> error1 1/1  "<z_Kg_dt>"

== system QuadcopterSimModel_INDI_Traj/Controller INDI/Multicopter INDI Loiter Flight Mode/Multicopter Altitude Hold Flight Mode with INDI and reduced attitude control/Multicopter Altitude INDI Controller1/measure ==
  z_Kg : Inport
  z_Kg_dt : Inport  Port=2
  z_Kg_dt2 : Inport  Port=3
  Bus Creator : BusCreator  Inputs=3
  measure : Outport
  wires:
  Bus Creator/1 -> measure/1  "measure"
  z_Kg_dt2/1 -> Bus Creator/3  "z_Kg_dt2"
  z_Kg_dt/1 -> Bus Creator/2  "z_Kg_dt"
  z_Kg/1 -> Bus Creator/1  "z_Kg"

== system QuadcopterSimModel_INDI_Traj/Controller INDI/Multicopter INDI Loiter Flight Mode/Multicopter Altitude Hold Flight Mode with INDI and reduced attitude control/Multicopter Altitude INDI Controller1/ny control ==
  error_alt : Inport
  Bus to Vector : BusToVector
  Gain : Gain  Gain=alt_cntrl.K  Multiplication=Matrix(K*u)
  ny_cntrl : Outport
  wires:
  Gain/1 -> ny_cntrl/1
  Bus to Vector/1 -> Gain/1
  error_alt/1 -> Bus to Vector/1

== system QuadcopterSimModel_INDI_Traj/Controller INDI/Multicopter INDI Loiter Flight Mode/Multicopter Altitude Hold Flight Mode with INDI and reduced attitude control/Multicopter Altitude INDI Controller1/ny from reference ==
  reference_alt : Inport
  Bus Selector2 : BusSelector  OutputSignals=z_Kg_dt2
  ny_ref : Outport
  wires:
  Bus Selector2/1 -> ny_ref/1  "<z_Kg_dt2>"
  reference_alt/1 -> Bus Selector2/1

== system QuadcopterSimModel_INDI_Traj/Controller INDI/Multicopter INDI Loiter Flight Mode/Multicopter Altitude Hold Flight Mode with INDI and reduced attitude control/Multicopter Altitude INDI Controller1/ny measured ==
  measures : Inport
  Bus Selector2 : BusSelector  OutputSignals=z_Kg_dt2
  ny_measure : Outport
  wires:
  measures/1 -> Bus Selector2/1
  Bus Selector2/1 -> ny_measure/1  "<z_Kg_dt2>"

== system QuadcopterSimModel_INDI_Traj/Controller INDI/Multicopter INDI Loiter Flight Mode/Multicopter Altitude Hold Flight Mode with INDI and reduced attitude control/Multicopter Altitude INDI Controller1/reference model ==
  cmd_throttle : Inport
  initial_altitude : Inport  Port=2
  manual_mode : Inport  Port=3
  1-D Lookup Table : Lookup_n-D  NumberOfTableDimensions=1  BreakpointsForDimension1=[-1,0,1]  Table=[alt_cntrl.rm.w.max_descend,0,-alt_cntrl.rm.w.max_climb]  InternalRulePriority=Speed  RndMeth=Simplest  InputSameDT=on
  Bus Creator1 : BusCreator  Inputs=3
  Bus Selector4 : BusSelector  OutputSignals=x_ref,x_dt_ref
  Discrete-Time Integrator3 : DiscreteIntegrator  ExternalReset=rising  InitialConditionSource=external  SampleTime=-1  ICPrevOutput=DiscIntNeverNeededParam  ICPrevScaledInput=DiscIntNeverNeededParam
  Gain1 : Gain
  Gain2 : Gain
  PT1 reference model : ndi_lib/PT1 reference model  T=alt_cntrl.rm.w.T  x_max=alt_cntrl.rm.w.dt_up  x_min=-alt_cntrl.rm.w.dt_down  x_dt_max=inf  x_dt_min=-inf  x_init=0
      settings: SourceProductName=LADAC
  reference : Outport
  wires:
  initial_altitude/1 -> Discrete-Time Integrator3/3  "initial height"
  Gain2/1 -> Bus Creator1/3  "z_Kg_dt2"
  Gain1/1 -> Bus Creator1/2  "z_Kg_dt"
  Discrete-Time Integrator3/1 -> Bus Creator1/1  "z_Kg"
  Bus Creator1/1 -> reference/1  "altitude"
  Bus Selector4/2 -> Gain2/1  "<x_dt_ref>"
  PT1 reference model/1 -> Bus Selector4/1
  Bus Selector4/1 -> Gain1/1, Discrete-Time Integrator3/1  "<x_ref>"
  cmd_throttle/1 -> 1-D Lookup Table/1
  1-D Lookup Table/1 -> PT1 reference model/1
  manual_mode/1 -> Discrete-Time Integrator3/2

== system QuadcopterSimModel_INDI_Traj/Controller INDI/Multicopter INDI Loiter Flight Mode/Waypoint Reference/waypoint Reference System/Subsystem2 ==
  r_cmd : Inport
  Demux : Demux  Outputs=3
  Selector : Selector  InputPortWidth=12  IndexOptions=Index vector (dialog)  Indices=1:4:12  OutputSizes=1
  Selector5 : Selector  InputPortWidth=12  IndexOptions=Index vector (dialog)  Indices=2:4:12  OutputSizes=1
  Selector6 : Selector  InputPortWidth=12  IndexOptions=Index vector (dialog)  Indices=3:4:12  OutputSizes=1
  Selector7 : Selector  InputPortWidth=12  IndexOptions=Index vector (dialog)  Indices=4:4:12  OutputSizes=1
  Terminator : Terminator
  Terminator1 : Terminator
  Terminator2 : Terminator
  Vector Concatenate : Concatenate  NumInputs=3
  n-th Order Filter1 : Subsystem  mask{order=5, omega=6, output_order=4, use_inital_value=on}
      mask prompts: order "Filter order"; omega "Filter omega"; output_order "Outout Order"; use_inital_value "Start steady-state"
      mask init:
      | ss_model.order = order;
      | ss_model.omega = omega;
      | 
      | ss_model.K = ndiFeedbackGainPlace( -ss_model.omega*ones(ss_model.order,1), 0)
      | ss_model.A = diag(ones(ss_model.order-1,1),1)
      | ss_model.A(ss_model.order,:) = -ss_model.K';
      | 
      | ss_model.B = zeros(ss_model.order);
      | ss_model.C = eye(ss_model.order);
      | ss_model.D = zeros(ss_model.order);
      | 
      | ss_model.B(ss_model.order,ss_model.order) = ss_model.K(1);
  n-th Order Filter2 : Subsystem  mask{order=5, omega=6, output_order=4, use_inital_value=on}
      mask prompts: order "Filter order"; omega "Filter omega"; output_order "Outout Order"; use_inital_value "Start steady-state"
      mask init: same as QuadcopterSimModel_INDI_Traj/Controller INDI/Multicopter INDI Loiter Flight Mode/Waypoint Reference/waypoint Reference System/Subsystem2/n-th Order Filter1
  n-th Order Filter3 : Subsystem  mask{order=5, omega=6, output_order=4, use_inital_value=on}
      mask prompts: order "Filter order"; omega "Filter omega"; output_order "Outout Order"; use_inital_value "Start steady-state"
      mask init: same as QuadcopterSimModel_INDI_Traj/Controller INDI/Multicopter INDI Loiter Flight Mode/Waypoint Reference/waypoint Reference System/Subsystem2/n-th Order Filter1
  r_r : Outport
  v_r : Outport  Port=2
  a_r : Outport  Port=3
  j_r : Outport  Port=4
  wires:
  Selector7/1 -> j_r/1
  Selector5/1 -> v_r/1
  r_cmd/1 -> Demux/1
  Selector/1 -> r_r/1
  Demux/1 -> n-th Order Filter2/1(w)
  n-th Order Filter3/1(y1) -> Terminator2/1
  n-th Order Filter2/1(y1) -> Terminator/1
  Selector6/1 -> a_r/1
  Demux/3 -> n-th Order Filter3/1(w)
  Demux/2 -> n-th Order Filter1/1(w)
  n-th Order Filter1/1(y1) -> Terminator1/1
  Vector Concatenate/1 -> Selector5/1, Selector/1, Selector7/1, Selector6/1
  n-th Order Filter2/3(y_out) -> Vector Concatenate/1
  n-th Order Filter3/3(y_out) -> Vector Concatenate/3
  n-th Order Filter1/3(y_out) -> Vector Concatenate/2

== system QuadcopterSimModel_INDI_Traj/Controller INDI/Multicopter INDI Loiter Flight Mode/Multicopter Altitude Hold Flight Mode with INDI and reduced attitude control/Multicopter (Reduced) Attitude INDI Controller/reference model/Subsystem ==
  <x_ref> : Inport
  PT2 discrete with saturation : Subsystem  mask{omega=2./T, d=1, x_dt2_max=inf, x_dt2_min=-inf, x_dt_max=inf, x_dt_min=-inf, x_max=inf, x_min=-inf, x_init=0, x_dt_init=0}
      mask prompts: omega "Natural frequency"; d "Damping ratio"; x_dt2_max "Maximum acceleration"; x_dt2_min "Minimum acceleration"; x_dt_max "Maximum rate"; x_dt_min "Minimum rate"; x_max "Maximum position"; x_min "Minimum position"; x_init "Initial position"; x_dt_init "Initial rate"
  Terminator : Terminator
  Terminator1 : Terminator
  Out1 : Outport
  wires:
  <x_ref>/1 -> PT2 discrete with saturation/1(u), PT2 discrete with saturation/2(u_0)
  PT2 discrete with saturation/1(y) -> Out1/1
  PT2 discrete with saturation/3(y_dt2) -> Terminator1/1
  PT2 discrete with saturation/2(y_dt) -> Terminator/1

== system QuadcopterSimModel_INDI_Traj/Controller INDI/Multicopter INDI Loiter Flight Mode/Waypoint Reference/waypoint Reference System/Subsystem2/n-th Order Filter1 ==
  w : Inport
  Add : Sum
  Assignment1 : Assignment  DiagnosticForDimensions=Warning  IndexOptions=Index vector (dialog)  Indices=ss_model.order  OutputSizes=1
  Assignment2 : Assignment  DiagnosticForDimensions=Warning  IndexOptions=Index vector (dialog)  Indices=1  OutputSizes=1
  Constant8 : Constant  Value=zeros(ss_model.order,1)  VectorParams1D=off
  Gain : Gain  Gain=ss_model.A  Multiplication=Matrix(K*u)
  Gain1 : Gain  Gain=ss_model.B  Multiplication=Matrix(K*u)
  Gain2 : Gain  Gain=ss_model.C  Multiplication=Matrix(K*u)
  Gain3 : Gain  Gain=use_inital_value
  Integrator : Integrator  InitialConditionSource=external
  Selector : Selector  InputPortWidth=ss_model.order  IndexOptions=Index vector (dialog)  Indices=1  OutputSizes=1
  Selector1 : Selector  InputPortWidth=ss_model.order  IndexOptions=Index vector (dialog)  Indices=1:output_order  OutputSizes=1
  y1 : Outport
  y_all : Outport  Port=2
  y_out : Outport  Port=3
  wires:
  Constant8/1 -> Assignment2/1, Assignment1/1
  w/1 -> Assignment2/2, Assignment1/2
  Selector/1 -> y1/1
  Integrator/1 -> Gain2/1, Gain/1
  Gain1/1 -> Add/1
  Assignment1/1 -> Gain1/1
  Add/1 -> Integrator/1
  Gain2/1 -> Selector1/1, y_all/1, Selector/1
  Gain/1 -> Add/2
  Assignment2/1 -> Gain3/1
  Gain3/1 -> Integrator/2
  Selector1/1 -> y_out/1

== system QuadcopterSimModel_INDI_Traj/Controller INDI/Multicopter INDI Loiter Flight Mode/Waypoint Reference/waypoint Reference System/Subsystem2/n-th Order Filter2 ==
  w : Inport
  Add : Sum
  Assignment1 : Assignment  DiagnosticForDimensions=Warning  IndexOptions=Index vector (dialog)  Indices=ss_model.order  OutputSizes=1
  Assignment2 : Assignment  DiagnosticForDimensions=Warning  IndexOptions=Index vector (dialog)  Indices=1  OutputSizes=1
  Constant8 : Constant  Value=zeros(ss_model.order,1)  VectorParams1D=off
  Gain : Gain  Gain=ss_model.A  Multiplication=Matrix(K*u)
  Gain1 : Gain  Gain=ss_model.B  Multiplication=Matrix(K*u)
  Gain2 : Gain  Gain=ss_model.C  Multiplication=Matrix(K*u)
  Gain3 : Gain  Gain=use_inital_value
  Integrator : Integrator  InitialConditionSource=external
  Selector : Selector  InputPortWidth=ss_model.order  IndexOptions=Index vector (dialog)  Indices=1  OutputSizes=1
  Selector1 : Selector  InputPortWidth=ss_model.order  IndexOptions=Index vector (dialog)  Indices=1:output_order  OutputSizes=1
  y1 : Outport
  y_all : Outport  Port=2
  y_out : Outport  Port=3
  wires:
  Constant8/1 -> Assignment2/1, Assignment1/1
  w/1 -> Assignment2/2, Assignment1/2
  Selector/1 -> y1/1
  Integrator/1 -> Gain2/1, Gain/1
  Gain1/1 -> Add/1
  Assignment1/1 -> Gain1/1
  Add/1 -> Integrator/1
  Gain2/1 -> Selector1/1, y_all/1, Selector/1
  Gain/1 -> Add/2
  Assignment2/1 -> Gain3/1
  Gain3/1 -> Integrator/2
  Selector1/1 -> y_out/1

== system QuadcopterSimModel_INDI_Traj/Controller INDI/Multicopter INDI Loiter Flight Mode/Waypoint Reference/waypoint Reference System/Subsystem2/n-th Order Filter3 ==
  w : Inport
  Add : Sum
  Assignment1 : Assignment  DiagnosticForDimensions=Warning  IndexOptions=Index vector (dialog)  Indices=ss_model.order  OutputSizes=1
  Assignment2 : Assignment  DiagnosticForDimensions=Warning  IndexOptions=Index vector (dialog)  Indices=1  OutputSizes=1
  Constant8 : Constant  Value=zeros(ss_model.order,1)  VectorParams1D=off
  Gain : Gain  Gain=ss_model.A  Multiplication=Matrix(K*u)
  Gain1 : Gain  Gain=ss_model.B  Multiplication=Matrix(K*u)
  Gain2 : Gain  Gain=ss_model.C  Multiplication=Matrix(K*u)
  Gain3 : Gain  Gain=use_inital_value
  Integrator : Integrator  InitialConditionSource=external
  Selector : Selector  InputPortWidth=ss_model.order  IndexOptions=Index vector (dialog)  Indices=1  OutputSizes=1
  Selector1 : Selector  InputPortWidth=ss_model.order  IndexOptions=Index vector (dialog)  Indices=1:output_order  OutputSizes=1
  y1 : Outport
  y_all : Outport  Port=2
  y_out : Outport  Port=3
  wires:
  Constant8/1 -> Assignment2/1, Assignment1/1
  w/1 -> Assignment2/2, Assignment1/2
  Selector/1 -> y1/1
  Integrator/1 -> Gain2/1, Gain/1
  Gain1/1 -> Add/1
  Assignment1/1 -> Gain1/1
  Add/1 -> Integrator/1
  Gain2/1 -> Selector1/1, y_all/1, Selector/1
  Gain/1 -> Add/2
  Assignment2/1 -> Gain3/1
  Gain3/1 -> Integrator/2
  Selector1/1 -> y_out/1

== system QuadcopterSimModel_INDI_Traj/Controller INDI/Multicopter INDI Loiter Flight Mode/Multicopter Altitude Hold Flight Mode with INDI and reduced attitude control/Multicopter (Reduced) Attitude INDI Controller/reference model/Subsystem/PT2 discrete with saturation ==
  u : Inport
  u_0 : Inport  Port=2
  2*d/omega : Gain  Gain=2*d./omega
  Discrete-Time Integrator y : DiscreteIntegrator  InitialConditionSource=external  InitialCondition=x_init  SampleTime=-1  OutDataTypeStr=Inherit: Inherit via back propagation  LimitOutput=on  UpperSaturationLimit=x_max  LowerSaturationLimit=x_min  ICPrevOutput=DiscIntNeverNeededParam  ICPrevScaledInput=DiscIntNeverNeededParam
  Discrete-Time Integrator y_dt : DiscreteIntegrator  InitialCondition=x_dt_init  SampleTime=-1  OutDataTypeStr=Inherit: Inherit via back propagation  LimitOutput=on  UpperSaturationLimit=x_dt_max  LowerSaturationLimit=x_dt_min  ICPrevOutput=DiscIntNeverNeededParam  ICPrevScaledInput=DiscIntNeverNeededParam
  Saturation : Saturate  UpperLimit=x_dt2_max  LowerLimit=x_dt2_min
  Sum2 : Sum  Inputs=|+-
  Sum3 : Sum  Inputs=|++
  omega^2 : Gain  Gain=omega.^2
  y : Outport
  y_dt : Outport  Port=2
  y_dt2 : Outport  Port=3
  wires:
  u_0/1 -> Discrete-Time Integrator y/2
  Discrete-Time Integrator y_dt/1 -> Discrete-Time Integrator y/1, y_dt/1, 2*d/omega/1  "y_dt"
  Discrete-Time Integrator y/1 -> y/1, Sum3/1  "y"
  Sum2/1 -> omega^2/1
  2*d/omega/1 -> Sum3/2
  u/1 -> Sum2/1
  Sum3/1 -> Sum2/2
  omega^2/1 -> Saturation/1
  Saturation/1 -> Discrete-Time Integrator y_dt/1, y_dt2/1  "y_dt2"

== matlab function QuadcopterSimModel_INDI_Traj/Controller INDI/Multicopter INDI Loiter Flight Mode/command direction/MATLAB Function ==
  data: cmd_u input; cmd_u_N output; cmd_v input; is_NED input; cmd_v_E output; M_bg input
function [cmd_u_N,cmd_v_E] = fcn( cmd_u, cmd_v, is_NED, M_bg )

if is_NED
    cmd_u_N = cmd_u;
    cmd_v_E = cmd_v;
else
    EulerAngle = dcm2Euler(M_bg);
    yaw = EulerAngle(3);
    M_NED_FRD = euler2Dcm([0;0;yaw])';
    cmd_V_NED = M_NED_FRD * [ cmd_u; cmd_v; 0 ];
    cmd_u_N = cmd_V_NED(1);
    cmd_v_E = cmd_V_NED(2);
end

end

== matlab function QuadcopterSimModel_INDI_Traj/Controller INDI/Multicopter INDI Loiter Flight Mode/Delta attitude to stick commands/conversion to total attitude command/MATLAB Function1 ==
  data: M_bg input; n_g output
function n_g = dcm2LeanVector( M_bg )
n_g = dcm2LeanVector( M_bg );
end

== matlab function QuadcopterSimModel_INDI_Traj/Controller INDI/Multicopter INDI Loiter Flight Mode/Delta attitude to stick commands/MATLAB Function1 ==
  data: lean_angle_0_1 input; stick_roll_cmd output; lean_direction_angle input; stick_pitch_cmd output
function [stick_roll_cmd,stick_pitch_cmd] = fcn(lean_angle_0_1,lean_direction_angle)

stick_roll_cmd = lean_angle_0_1 * sin( lean_direction_angle );
stick_pitch_cmd = - lean_angle_0_1 * cos( lean_direction_angle );

end

== matlab function QuadcopterSimModel_INDI_Traj/Controller INDI/Multicopter INDI Loiter Flight Mode/Horizontal NDI position (NE) controller cascade with reduced attitude (angle) command/filtered command/MATLAB Function1 ==
  data: stick_roll_cmd input; cmd_velocity_abs_0_1 output; stick_pitch_cmd input; lean_direction_angle output
function [cmd_velocity_abs_0_1,lean_direction_angle] = fcn(stick_roll_cmd,stick_pitch_cmd)

lean_direction_angle = atan2(stick_roll_cmd,-stick_pitch_cmd);
cmd_velocity_abs_0_1 = sqrt( stick_roll_cmd^2 + stick_pitch_cmd^2 );

end

== matlab function QuadcopterSimModel_INDI_Traj/Controller INDI/Multicopter INDI Loiter Flight Mode/Horizontal NDI position (NE) controller cascade with reduced attitude (angle) command/Convert to reduced attitude pseudo control/MATLAB Function2 ==
  data: phi output; delta output; xyz_g_dt2 input
function [phi,delta] = fcn(xyz_g_dt2)
% function [x,y] = fcn(xyz_g_dt2)

if abs(xyz_g_dt2(3)) < 1
    if xyz_g_dt2(3) > 0
        xyz_g_dt2(3) = 1;
    else
        xyz_g_dt2(3) = -1;
    end
end

% x = atan2(xyz_g_dt2(1),-xyz_g_dt2(3));
% y = atan2(xyz_g_dt2(2),-xyz_g_dt2(3));


delta = atan2(xyz_g_dt2(2),xyz_g_dt2(1));
xy_g_dt2 = sqrt( xyz_g_dt2(1)^2 + xyz_g_dt2(2)^2 );
phi = atan2( xy_g_dt2 , -xyz_g_dt2(3) );

end

== matlab function QuadcopterSimModel_INDI_Traj/Controller INDI/Multicopter INDI Loiter Flight Mode/Horizontal NDI position (NE) controller cascade with reduced attitude (angle) command/Convert to reduced attitude pseudo control/MATLAB Function3 ==
  data: q_cmd_red output; phi input; delta input
function q_cmd_red  = fcn(phi,delta)

x = sin(delta);
y = -cos(delta);

xy = sqrt(x^2+y^2);
if xy <= 1e-2
    x = single(1);
    xy_save = sqrt(x^2+y^2);
else
    xy_save = xy;
end
n_d_red = 1/xy_save*[x;y;0];

% [1] eq. (1)
q_0 = cos(phi/2);
q_t = n_d_red * sin(phi/2);
q_cmd_red = [q_0;q_t];

end

== matlab function QuadcopterSimModel_INDI_Traj/Controller INDI/Multicopter INDI Loiter Flight Mode/Multicopter Altitude Hold Flight Mode with INDI and reduced attitude control/MATLAB Function ==
  data: u input; y output
function y = fcn(u)
y = 0.5*u+0.5;

== matlab function QuadcopterSimModel_INDI_Traj/Controller INDI/Multicopter INDI Loiter Flight Mode/Horizontal NDI position (NE) controller cascade with reduced attitude (angle) command/Convert to reduced attitude pseudo control/MATLAB Function8 ==
  data: q_cmd_red output; phi input; delta input
function q_cmd_red  = fcn(phi,delta)

x = sin(delta);
y = -cos(delta);

xy = sqrt(x^2+y^2);
if xy <= 1e-2
    x = single(1);
    xy_save = sqrt(x^2+y^2);
else
    xy_save = xy;
end
n_d_red = 1/xy_save*[x;y;0];

% [1] eq. (1)
q_0 = cos(phi/2);
q_t = n_d_red * sin(phi/2);
q_cmd_red = [q_0;q_t];

end

== matlab function QuadcopterSimModel_INDI_Traj/Controller INDI/Multicopter INDI Loiter Flight Mode/Multicopter Altitude Hold Flight Mode with INDI and reduced attitude control/MATLAB Function1 ==
  data: stick_roll_cmd input; lean_angle output; stick_pitch_cmd input; lean_direction_angle output
function [lean_angle,lean_direction_angle] = fcn(stick_roll_cmd,stick_pitch_cmd)

lean_direction_angle = atan2(stick_roll_cmd,-stick_pitch_cmd);
lean_angle = sqrt( stick_roll_cmd^2 + stick_pitch_cmd^2 );

end

== matlab function QuadcopterSimModel_INDI_Traj/Controller INDI/Multicopter INDI Loiter Flight Mode/Multicopter Altitude Hold Flight Mode with INDI and reduced attitude control/acceleration g to b frame/MATLAB Function ==
  data: z_Kg_dt2_cmd input; z_Kb_dt2_cmd output; lean_angle input
function z_Kb_dt2_cmd = fcn(z_Kg_dt2_cmd,lean_angle)

% compensate lean angle
cos_lean = cos(lean_angle);
if cos_lean > 0.1
    z_Kb_dt2_cmd = z_Kg_dt2_cmd / cos_lean;
else
    z_Kb_dt2_cmd = z_Kg_dt2_cmd;
end

end

== matlab function QuadcopterSimModel_INDI_Traj/Controller INDI/Multicopter INDI Loiter Flight Mode/Multicopter Altitude Hold Flight Mode with INDI and reduced attitude control/acceleration g to b frame/dcm2Lean ==
  data: M_bg input; phi output
function phi= dcm2Lean( M_bg )
[phi,~] = dcm2Lean( M_bg );
end
